simulink model "Simul_ContPID"  (R2024b)
settings: Solver=VariableStepAuto  StartTime=0.0  StopTime=6  RelTol=1e-3
undefined symbols (not defined in the file): T
settings Model: Creator=Celso  LastModifiedBy=syaba

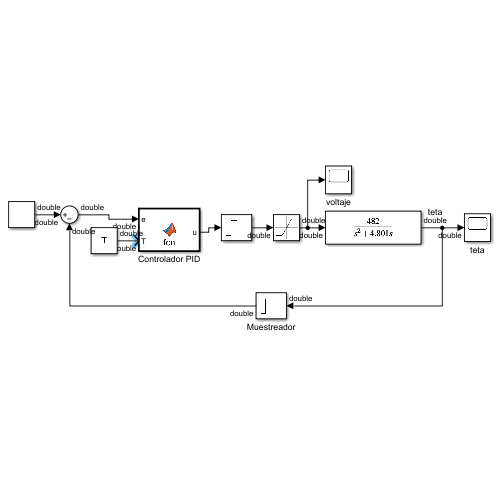
[thumbnail: Simulink's stored preview of the top-level diagram]
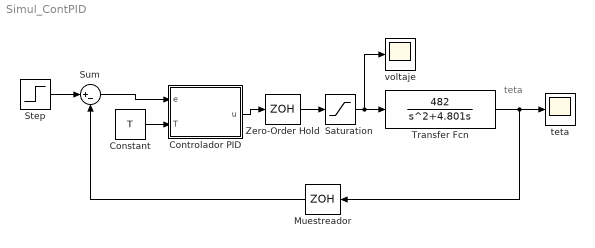
== system Simul_ContPID ==
  note: teta
  Constant : Constant  Value=T
  Controlador PID : MATLAB Function  TreatAsAtomicUnit=on  SystemSampleTime=T
  Muestreador : ZeroOrderHold  SampleTime=T
  Saturation : Saturate  UpperLimit=3  LowerLimit=-3
  Step : Step  Time=0  After=100  SampleTime=T
  Sum : Sum  Inputs=|+-
  Transfer Fcn : TransferFcn  Numerator=[482]  Denominator="[1 4.801  0]"
  Zero-Order Hold : ZeroOrderHold  SampleTime=T
  teta : Scope
  voltaje : Scope
  wires:
  Constant/1 -> Controlador PID/2(T)
  Sum/1 -> Controlador PID/1(e)
  Step/1 -> Sum/1
  Controlador PID/1(u) -> Zero-Order Hold/1
  Transfer Fcn/1 -> teta/1, Muestreador/1
  Muestreador/1 -> Sum/2
  Zero-Order Hold/1 -> Saturation/1
  Saturation/1 -> voltaje/1, Transfer Fcn/1

== matlab function Simul_ContPID/Controlador PID ==
  data: e input; u output; T input
function u = fcn(e,T)

Kp=0.0669;
Td=0.25;
Ti=1;

persistent e_ant;
persistent I_ant;

if isempty(e_ant),
    e_ant=0;
end;

if isempty(I_ant),
    I_ant=0;
end;


D = (e-e_ant)/T;
I = I_ant + e*T;


u = Kp*(e+ (1/Ti)*I + Td*D);

e_ant = e;
I_ant = I;
